simulink model "lorenzs"  (Simulink 6.0)
settings: Solver=ode23  SolverMode=SingleTasking  StartTime=0.0  StopTime=inf  RelTol=1e-3  AbsTol=1e-6
libraries: simulink x1
settings Model: Creator=The MathWorks Inc.  LastModifiedBy=batserve  ExtModeTrigMode=oneshot  ExtModeArmWhenConnect=off  ExtModeAutoUpdateStatusClock=off
settings DataIOCC: ExternalInput=[]  InitialState=[]  LimitDataPoints=off  SaveOutput=off  SaveTime=off
settings OptimizationCC: BooleanDataType=off
settings DebuggingCC: CheckExecutionContextPreStartOutputMsg=on  CheckExecutionContextRuntimeOutputMsg=on  SolverPrmCheckMsg=none  IntegerOverflowMsg=none
settings HardwareCC: TargetUnknown=on

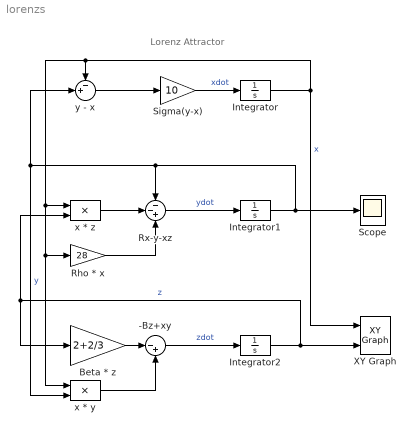
== system lorenzs ==
  note: Lorenz Attractor
  -Bz+xy : Sum  Inputs=|-+  SaturateOnIntegerOverflow=on  InputSameDT=on
  Beta * z : Gain  Gain=2+2/3  SaturateOnIntegerOverflow=on
  Integrator : Integrator  InitialCondition=1
  Integrator1 : Integrator  InitialCondition=1
  Integrator2 : Integrator  InitialCondition=1
  Rho * x : Gain  Gain=28  SaturateOnIntegerOverflow=on
  Rx-y-xz : Sum  Inputs=--+  SaturateOnIntegerOverflow=on  InputSameDT=on
  Scope : Scope
      settings: TickLabels=on  TimeRange=20  YMin=-25  YMax=30  DataFormat=Array
  Sigma(y-x) : Gain  Gain=10  SaturateOnIntegerOverflow=on
  XY Graph : simulink/Sinks/XY Graph  xmin=-30  xmax=30  ymin=0  ymax=50  st=-1
  x * y : Product  SaturateOnIntegerOverflow=on  RndMeth=Zero  InputSameDT=on
  x * z : Product  SaturateOnIntegerOverflow=on  RndMeth=Zero  InputSameDT=on
  y - x : Sum  Inputs=-+|  SaturateOnIntegerOverflow=on  InputSameDT=on
  wires:
  Sigma(y-x)/1 -> Integrator/1  "xdot"
  y - x/1 -> Sigma(y-x)/1
  Rx-y-xz/1 -> Integrator1/1  "ydot"
  Rho * x/1 -> Rx-y-xz/3
  x * z/1 -> Rx-y-xz/2
  Integrator2/1 -> XY Graph/2, x * z/2, Beta * z/1  "z"
  Integrator1/1 -> Scope/1, Rx-y-xz/1, y - x/2, x * y/2  "y"
  Integrator/1 -> XY Graph/1, y - x/1, x * z/1, Rho * x/1, x * y/1  "x"
  -Bz+xy/1 -> Integrator2/1  "zdot"
  Beta * z/1 -> -Bz+xy/1
  x * y/1 -> -Bz+xy/2
